simulink model "ysw5_13"  (R2014a)
settings: Solver=ode45  StartTime=0.0  StopTime=10.0  RelTol=1e-3
settings Model: Creator=Administrator  LastModifiedBy=Administrator

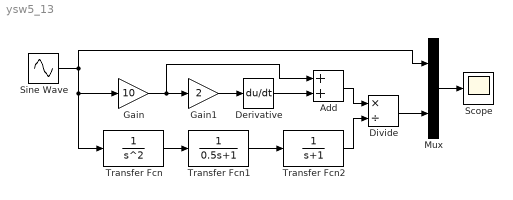
== system ysw5_13 ==
  Add : Sum
  Derivative : Derivative
  Divide : Product  Inputs=*/
  Gain : Gain  Gain=10
  Gain1 : Gain  Gain=2
  Mux : Mux  Inputs=2
  Scope : Scope
  Sine Wave : Sin  SampleTime=0
  Transfer Fcn : TransferFcn  Denominator=[1 0 0]
  Transfer Fcn1 : TransferFcn  Denominator=[0.5 1]
  Transfer Fcn2 : TransferFcn  Denominator=[1 1]
  wires:
  Sine Wave/1 -> Mux/1, Transfer Fcn/1, Gain/1
  Transfer Fcn1/1 -> Transfer Fcn2/1
  Transfer Fcn/1 -> Transfer Fcn1/1
  Mux/1 -> Scope/1
  Gain/1 -> Add/1, Gain1/1
  Gain1/1 -> Derivative/1
  Derivative/1 -> Add/2
  Add/1 -> Divide/1
  Transfer Fcn2/1 -> Divide/2
  Divide/1 -> Mux/2
